simulink model "unitVisualAqSurveillance"  (R2019b)
settings: Solver=VariableStepAuto  StartTime=0.0  StopTime=10.0  RelTol=1e-3
undefined symbols (not defined in the file or in its folder): ac1dyn_alt0_ft, ac1dyn_con, ac1dyn_lat0_rad, ac1dyn_lon0_rad, ac2dyn_alt0_ft, ac2dyn_con, ac2dyn_lat0_rad, ac2dyn_lon0_rad, ddh_ftps2, dh_ftps, dv_ftps2, e_ft, Edot_ftps, h_ft, hdot_ftps, latLonAltState, n_ft, Ndot_ftps, p_radps, phi_rad, phidot_radps, psi_rad, psidot_radps, q_radps, r_radps, theta_rad, thetadot_radps, v_ftps, vdot_fpss
libraries: simulink x14, VisualAqSurveillanceBlock_devAlt x1
(part 1 of 2)
settings Model: Creator=PE29732  LastModifiedBy=ng21251
settings DataIOCC: ReturnWorkspaceOutputs=off
settings DebuggingCC: ArithmeticOperatorsInVariantConditions=warning
settings SFSimCC: CustomCodeUndefinedFunction=UseInterfaceOnly

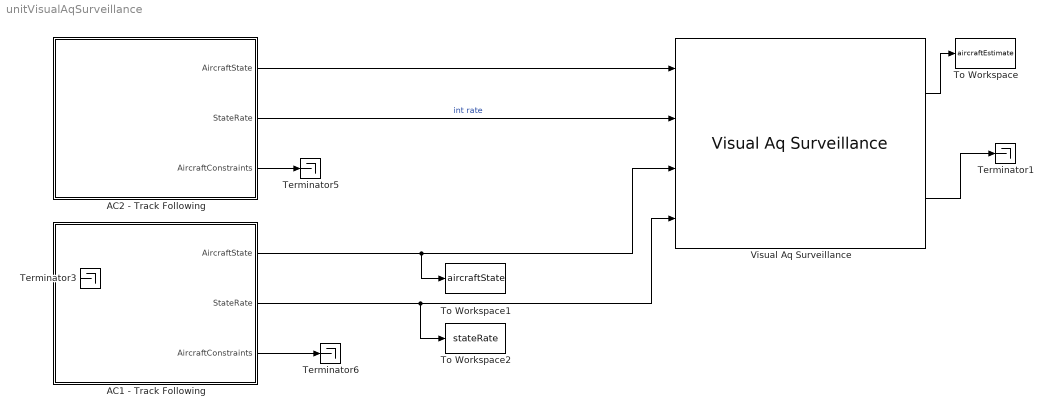
== system unitVisualAqSurveillance ==
  AC1 - Track Following : Subsystem  mask(Basic Aircraft Dynamic Model){ts_dynamics=0.1, lat0_rad=ac1dyn_lat0_rad, lon0_rad=ac1dyn_lon0_rad, alt_ft=ac1dyn_alt0_ft, v_ftps_max=ac1dyn_con.maxAirspeed_ftps, v_ftps_min=ac1dyn_con.minAirspeed_ftps, dv_ftpss_max=ac1dyn_con.maxAcceleration_ftpss, dv_ftpss_min=ac1dyn_con.minAcceleration_ftpss, dh_ftps_max=ac1dyn_con.maxVerticalRate_ftps, dh_ftps_min=ac1dyn_con.minVerticalRate_ftps, q_radps_max=ac1dyn_con.maxPitchRate_radps, phi_rad_max=ac1dyn_con.maxBankAngle_rad, dphi_radps_max=ac1dyn_con.maxRollRate_radps, r_radps_max=ac1dyn_con.maxYawRate_radps, pNUM=ac1dyn_con.dynamicsNumeratorRollRate, pDEN=ac1dyn_con.dynamicsDenominatorRollRate, hNUM=ac1dyn_con.dynamicsNumeratorVerticalRate, hDEN=ac1dyn_con.dynamicsDenominatorVerticalRate, rNUM=ac1dyn_con.dynamicsNumeratorYawRate, rDEN=ac1dyn_con.dynamicsDenominatorYawRate}
      mask prompts: ts_dynamics "Dynamics update parameter"; lat0_rad "Latitude of ENU origin (rad)"; lon0_rad "Longitude of ENU origin (rad)"; alt_ft "Height of ENU origin (ft)"; v_ftps_max "Maximum airspeed (ft/s)"; v_ftps_min "Minimum airspeed (ft/s)"; dv_ftpss_max "Maximum acceleration (ft/s/s)"; dv_ftpss_min "Miniimum acceleration (ft/s/s)"; dh_ftps_max "Maximum vertical rate (ft/s)"; dh_ftps_min "Minimum vertical rate (ft/s)"; q_radps_max "Maximum pitch rate (rad/s)"; phi_rad_max "Maximum bank angle (rad)"; dphi_radps_max "Maximum roll rate (rad/s)"; r_radps_max "Maximum yaw rate (rad/s)"; pNUM "Roll rate discrete dynamics numerator (2x1)"; pDEN "Roll rate discrete dynamics denominator (1x1)"; hNUM "Vertical rate discrete dynamics numerator (2x1)"; hDEN "Vertical rate discrete dynamics denominator (1x1)"; rNUM "Yaw rate discrete dynamics numerator (2x1)"; rDEN "Yaw rate discrete dynamics denominator (1x1)"
      mask help:
      | Propagates the aircraft dynamics using 6DOF equations of motion.
      |
      | The class Simple6DOF can be used to programmatically set the parameters of Basic Aircraft Dynamcis blocks.
      mask Help:
      | Propagates the aircraft dynamics using 6DOF equations of motion.
      | 
      | The class Simple6DOF can be used to programmatically set the parameters of Basic Aircraft Dynamcis blocks.
      mask DialogControl ParameterTabVar0 Prompt: Main
      mask DialogControl ParameterTabVar01 Prompt: Constraints
  AC2 - Track Following : Subsystem  mask(Basic Aircraft Dynamic Model){ts_dynamics=0.1, lat0_rad=ac2dyn_lat0_rad, lon0_rad=ac2dyn_lon0_rad, alt_ft=ac2dyn_alt0_ft, v_ftps_max=ac2dyn_con.maxAirspeed_ftps, v_ftps_min=ac2dyn_con.minAirspeed_ftps, dv_ftpss_max=ac2dyn_con.maxAcceleration_ftpss, dv_ftpss_min=ac2dyn_con.minAcceleration_ftpss, dh_ftps_max=ac2dyn_con.maxVerticalRate_ftps, dh_ftps_min=ac2dyn_con.minVerticalRate_ftps, q_radps_max=ac2dyn_con.maxPitchRate_radps, phi_rad_max=ac2dyn_con.maxBankAngle_rad, dphi_radps_max=ac2dyn_con.maxRollRate_radps, r_radps_max=ac2dyn_con.maxYawRate_radps, pNUM=ac2dyn_con.dynamicsNumeratorRollRate, pDEN=ac2dyn_con.dynamicsDenominatorRollRate, hNUM=ac2dyn_con.dynamicsNumeratorVerticalRate, hDEN=ac2dyn_con.dynamicsDenominatorVerticalRate, rNUM=ac2dyn_con.dynamicsNumeratorYawRate, rDEN=ac2dyn_con.dynamicsDenominatorYawRate}
      mask prompts: ts_dynamics "Dynamics update parameter"; lat0_rad "Latitude of ENU origin (rad)"; lon0_rad "Longitude of ENU origin (rad)"; alt_ft "Height of ENU origin (ft)"; v_ftps_max "Maximum airspeed (ft/s)"; v_ftps_min "Minimum airspeed (ft/s)"; dv_ftpss_max "Maximum acceleration (ft/s/s)"; dv_ftpss_min "Miniimum acceleration (ft/s/s)"; dh_ftps_max "Maximum vertical rate (ft/s)"; dh_ftps_min "Minimum vertical rate (ft/s)"; q_radps_max "Maximum pitch rate (rad/s)"; phi_rad_max "Maximum bank angle (rad)"; dphi_radps_max "Maximum roll rate (rad/s)"; r_radps_max "Maximum yaw rate (rad/s)"; pNUM "Roll rate discrete dynamics numerator (2x1)"; pDEN "Roll rate discrete dynamics denominator (1x1)"; hNUM "Vertical rate discrete dynamics numerator (2x1)"; hDEN "Vertical rate discrete dynamics denominator (1x1)"; rNUM "Yaw rate discrete dynamics numerator (2x1)"; rDEN "Yaw rate discrete dynamics denominator (1x1)"
      mask help:
      | Propagates the aircraft dynamics using 6DOF equations of motion.
      |
      | The class Simple6DOF can be used to programmatically set the parameters of Basic Aircraft Dynamcis blocks.
      mask Help:
      | Propagates the aircraft dynamics using 6DOF equations of motion.
      | 
      | The class Simple6DOF can be used to programmatically set the parameters of Basic Aircraft Dynamcis blocks.
      mask DialogControl ParameterTabVar0 Prompt: Main
      mask DialogControl ParameterTabVar01 Prompt: Constraints
  Terminator{1,3,5..6} (4 alike) : Terminator
  To Workspace : ToWorkspace  VariableName=aircraftEstimate  SaveFormat=Timeseries  SampleTime=-1
  To Workspace1 : ToWorkspace  VariableName=aircraftState  SaveFormat=Timeseries  SampleTime=-1
  To Workspace2 : ToWorkspace  VariableName=stateRate  SaveFormat=Timeseries  SampleTime=-1
  Visual Aq Surveillance : VisualAqSurveillanceBlock_devAlt/Visual Aq Surveillance  Description=|  dt=0.1
      | Documentation for Perfect Observation Block                                                                                                                                                                                                                                                                                                                                                                                                          
      |                                                                                                                                                                                                                                                                                                                                                                                                                                                      
      | Description:  The perfect observation block, also known as a perfect                                                                                                                                                                                                                                                                                                                                                                                 
      | surveillance block, receives an Aircraft State, nominally from a Basic                                                                                                                                                                                                                                                                                                                                                                               
      | Aircraft Dynamics block, and outputs an Aircraft Estimate.  The Aircraft                                                                                                                                                                                                                                                                                                                                                                             
      | State that is received as input consists of Latitude, Longitude, and                                                                                                                                                                                                                                                                                                                                                                                 
      | Altitude state information as well as the aircraft position in local                                                                                                                                                                                                                                                                                                                                                                                 
      | coordinates in units of feet for north, east, and height.  The Aircraft                                                                                                                                                                                                                                                                                                                                                                              
      | Estimate outputs consist of estimates for the aircraft Latitude, Longitude, and Altitude, the east, north up position, and sensor covariance.  For perfect surveillance, the covariance estimates are all set to zero as default.  In addition, "time of validity" and a Boolean flag for the sensor report, "is Valid", are outputted as part of the Aircraft Estimate.                                                                             
      |                                                                                                                                                                                                                                                                                                                                                                                                                                                      
      | The initial perfect surveillance block developed receives the aircraft state information from the "AC2 - Basic Aircraft Dynamics" block within the "nominalEncounter" study.  Since the expected output from the AC1 and AC2 aircraft states have slightly different output parameters than what is provided from the perfect surveillance block (i.e., covariance estimates, isValid, and time of validity), the perfect surveillance block         
      | AircraftEstimate output has been left disconnected.                                                                                                                                                                                                                                                                                                                                                                                                  
      |                                                                                                                                                                                                                                                                                                                                                                                                                                                      
      | The initial unit test performed for this perfect observation block was to                                                                                                                                                                                                                                                                                                                                                                            
      | run the nominalEncounter study and to ensure that the simulation completes and no exceptions are encountered.  This unit test was successful (other than receiving a warning that the output of the perfect surveillance block is not connected, which was expected).  A more comprehensive future unit test would be to evaluate the position inputs and compare them with the position outputs to ensure that they are consistent with one another.
  wires:
  AC1 - Track Following/1(AircraftState) -> Visual Aq Surveillance/3, To Workspace1/1
  Visual Aq Surveillance/1 -> To Workspace/1
  Visual Aq Surveillance/2 -> Terminator1/1
  AC1 - Track Following/2(StateRate) -> Visual Aq Surveillance/4, To Workspace2/1
  AC2 - Track Following/1(AircraftState) -> Visual Aq Surveillance/1
  AC2 - Track Following/3(AircraftConstraints) -> Terminator5/1
  AC1 - Track Following/3(AircraftConstraints) -> Terminator6/1
  AC2 - Track Following/2(StateRate) -> Visual Aq Surveillance/2  "int rate"

== system unitVisualAqSurveillance/AC1 - Track Following ==
  Follow Trajectory : Subsystem  mask(Follow Trajectory){trajfile=traj1.mat}
      mask prompts: trajfile "Trajectory File Name:"
      mask help: Reads trajectory data (North-East-Altitude position and velocity) from specified file. Computes other state variables to follow that trajectory. Ouptuts AircraftState and AircraftStateRate buses.
      mask init:
      | set_param( [ gcb '/Get Trajectory Data/From File' ], 'Filename', trajfile )
  Performance_constraints : Subsystem
  Rate Transition : RateTransition  OutPortSampleTime=0.1
  AircraftState : Outport  OutDataTypeStr=Bus: AircraftState  VectorParamsAs1DForOutWhenUnconnected=off
  StateRate : Outport  Port=2  OutDataTypeStr=Bus: AircraftStateRate  VectorParamsAs1DForOutWhenUnconnected=off
  AircraftConstraints : Outport  Port=3  OutDataTypeStr=Bus: AircraftConstraints  VectorParamsAs1DForOutWhenUnconnected=off
  wires:
  Follow Trajectory/2(State Rate) -> Rate Transition/1
  Follow Trajectory/1(State) -> AircraftState/1
  Performance_constraints/1(AircraftConstraints) -> Follow Trajectory/1(Constraints), AircraftConstraints/1
  Rate Transition/1 -> StateRate/1

== system unitVisualAqSurveillance/AC2 - Track Following ==
  Follow Trajectory : Subsystem  mask(Follow Trajectory){trajfile=traj2.mat}
      mask prompts: trajfile "Trajectory File Name:"
      mask help: Reads trajectory data (North-East-Altitude position and velocity) from specified file. Computes other state variables to follow that trajectory. Ouptuts AircraftState and AircraftStateRate buses.
      mask init:
      | set_param( [ gcb '/Get Trajectory Data/From File' ], 'Filename', trajfile )
  Performance_constraints : Subsystem
  Rate Transition : RateTransition  OutPortSampleTime=0.1
  AircraftState : Outport  OutDataTypeStr=Bus: AircraftState  VectorParamsAs1DForOutWhenUnconnected=off
  StateRate : Outport  Port=2  OutDataTypeStr=Bus: AircraftStateRate  VectorParamsAs1DForOutWhenUnconnected=off
  AircraftConstraints : Outport  Port=3  OutDataTypeStr=Bus: AircraftConstraints  VectorParamsAs1DForOutWhenUnconnected=off
  wires:
  Follow Trajectory/2(State Rate) -> Rate Transition/1
  Follow Trajectory/1(State) -> AircraftState/1
  Performance_constraints/1(AircraftConstraints) -> Follow Trajectory/1(Constraints), AircraftConstraints/1
  Rate Transition/1 -> StateRate/1

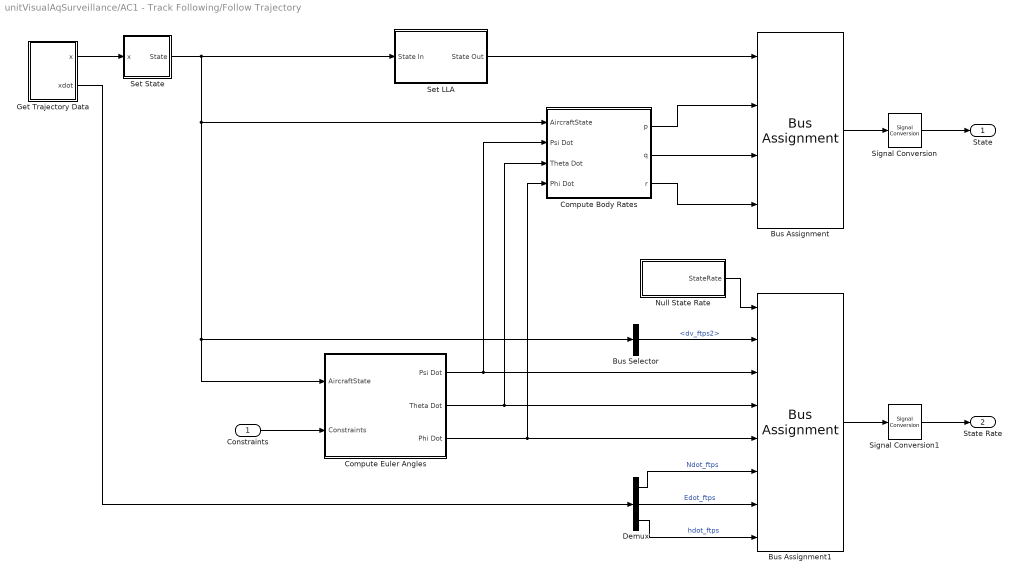
== system unitVisualAqSurveillance/AC1 - Track Following/Follow Trajectory ==
  Constraints : Inport
  Bus Assignment : BusAssignment  AssignedSignals=p_radps,q_radps,r_radps
  Bus Assignment1 : BusAssignment  AssignedSignals=vdot_fpss,psidot_radps,thetadot_radps,phidot_radps,Ndot_ftps,Edot_ftps,hdot_ftps
  Bus Selector : BusSelector  OutputSignals=dv_ftps2
  Compute Body Rates : Subsystem
  Compute Euler Angles : Subsystem
  Demux : Demux  Outputs=3
  Get Trajectory Data : Subsystem
  Null State Rate : Subsystem
  "Set LLA " : Subsystem  mask{lat0=lat0_rad, lon0=lon0_rad, h0=alt_ft}
      mask prompts: lat0 "ENU latitude origin (rad)"; lon0 "ENU longitude origin (rad)"; h0 "ENU altitude origin (ft)"
  Set State : Subsystem
  Signal Conversion : SignalConversion  OverrideOpt=off
  Signal Conversion1 : SignalConversion  OverrideOpt=off
  State : Outport  VectorParamsAs1DForOutWhenUnconnected=off
  State Rate : Outport  Port=2  VectorParamsAs1DForOutWhenUnconnected=off
  wires:
  Signal Conversion1/1 -> State Rate/1
  Bus Selector/1 -> Bus Assignment1/2  "<dv_ftps2>"
  Compute Euler Angles/3("Phi Dot ") -> Bus Assignment1/5, Compute Body Rates/4(Phi Dot)
  Compute Euler Angles/1(Psi Dot) -> Bus Assignment1/3, Compute Body Rates/2(Psi Dot)
  Demux/3 -> Bus Assignment1/8  "hdot_ftps"
  Null State Rate/1(StateRate) -> Bus Assignment1/1
  Get Trajectory Data/2(xdot) -> Demux/1
  Compute Body Rates/3(r) -> Bus Assignment/4
  Compute Body Rates/2(q) -> Bus Assignment/3
  Compute Body Rates/1(p) -> Bus Assignment/2
  Demux/1 -> Bus Assignment1/6  "Ndot_ftps"
  Demux/2 -> Bus Assignment1/7  "Edot_ftps"
  Compute Euler Angles/2(Theta Dot) -> Bus Assignment1/4, Compute Body Rates/3(Theta Dot)
  Signal Conversion/1 -> State/1
  "Set LLA "/1(State Out) -> Bus Assignment/1
  Bus Assignment/1 -> Signal Conversion/1
  Bus Assignment1/1 -> Signal Conversion1/1
  Set State/1(State) -> Compute Body Rates/1(AircraftState), Compute Euler Angles/1(AircraftState), Bus Selector/1, "Set LLA "/1(State In)
  Constraints/1 -> Compute Euler Angles/2(Constraints)
  Get Trajectory Data/1(x) -> Set State/1(x)

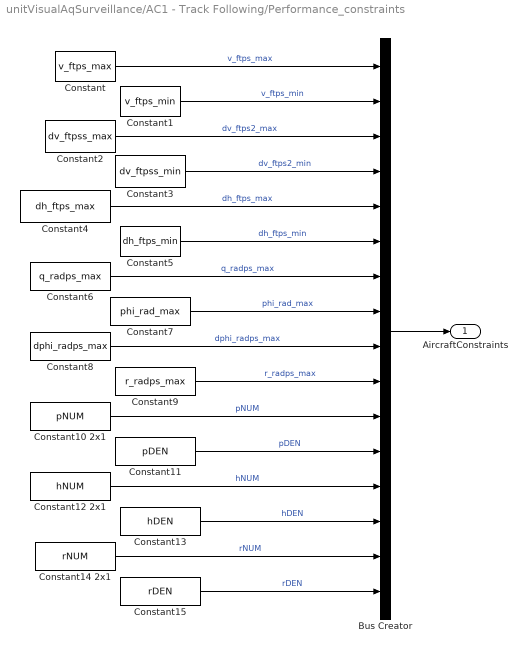
== system unitVisualAqSurveillance/AC1 - Track Following/Performance_constraints ==
  Bus Creator : BusCreator  Inputs=16
  Constant : Constant  Value=v_ftps_max
  Constant1 : Constant  Value=v_ftps_min
  Constant10 2x1 : Constant  Value=pNUM
  Constant11 : Constant  Value=pDEN
  Constant12 2x1 : Constant  Value=hNUM
  Constant13 : Constant  Value=hDEN
  Constant14 2x1 : Constant  Value=rNUM
  Constant15 : Constant  Value=rDEN
  Constant2 : Constant  Value=dv_ftpss_max
  Constant3 : Constant  Value=dv_ftpss_min
  Constant4 : Constant  Value=dh_ftps_max
  Constant5 : Constant  Value=dh_ftps_min
  Constant6 : Constant  Value=q_radps_max
  Constant7 : Constant  Value=phi_rad_max
  Constant8 : Constant  Value=dphi_radps_max
  Constant9 : Constant  Value=r_radps_max
  AircraftConstraints : Outport  OutDataTypeStr=Bus: AircraftConstraints  VectorParamsAs1DForOutWhenUnconnected=off
  wires:
  Constant10 2x1/1 -> Bus Creator/11  "pNUM"
  Constant12 2x1/1 -> Bus Creator/13  "hNUM"
  Constant14 2x1/1 -> Bus Creator/15  "rNUM"
  Constant8/1 -> Bus Creator/9  "dphi_radps_max"
  Constant7/1 -> Bus Creator/8  "phi_rad_max"
  Constant6/1 -> Bus Creator/7  "q_radps_max"
  Constant5/1 -> Bus Creator/6  "dh_ftps_min"
  Constant4/1 -> Bus Creator/5  "dh_ftps_max"
  Constant3/1 -> Bus Creator/4  "dv_ftps2_min"
  Constant2/1 -> Bus Creator/3  "dv_ftps2_max"
  Constant1/1 -> Bus Creator/2  "v_ftps_min"
  Constant/1 -> Bus Creator/1  "v_ftps_max"
  Bus Creator/1 -> AircraftConstraints/1
  Constant15/1 -> Bus Creator/16  "rDEN"
  Constant13/1 -> Bus Creator/14  "hDEN"
  Constant11/1 -> Bus Creator/12  "pDEN"
  Constant9/1 -> Bus Creator/10  "r_radps_max"

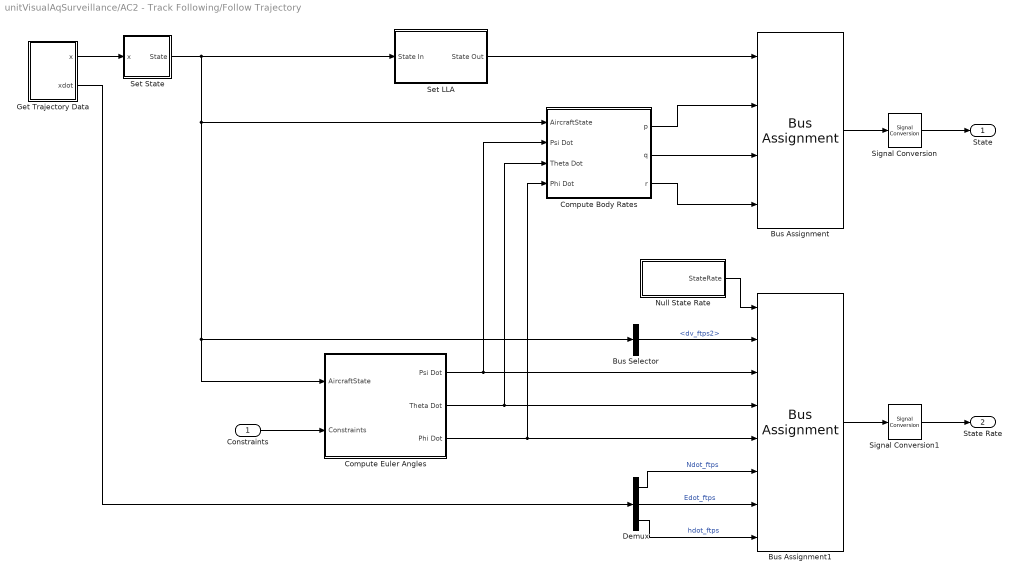
== system unitVisualAqSurveillance/AC2 - Track Following/Follow Trajectory ==
  Constraints : Inport
  Bus Assignment : BusAssignment  AssignedSignals=p_radps,q_radps,r_radps
  Bus Assignment1 : BusAssignment  AssignedSignals=vdot_fpss,psidot_radps,thetadot_radps,phidot_radps,Ndot_ftps,Edot_ftps,hdot_ftps
  Bus Selector : BusSelector  OutputSignals=dv_ftps2
  Compute Body Rates : Subsystem
  Compute Euler Angles : Subsystem
  Demux : Demux  Outputs=3
  Get Trajectory Data : Subsystem
  Null State Rate : Subsystem
  "Set LLA " : Subsystem  mask{lat0=lat0_rad, lon0=lon0_rad, h0=alt_ft}
      mask prompts: lat0 "ENU latitude origin (rad)"; lon0 "ENU longitude origin (rad)"; h0 "ENU altitude origin (ft)"
  Set State : Subsystem
  Signal Conversion : SignalConversion  OverrideOpt=off
  Signal Conversion1 : SignalConversion  OverrideOpt=off
  State : Outport  VectorParamsAs1DForOutWhenUnconnected=off
  State Rate : Outport  Port=2  VectorParamsAs1DForOutWhenUnconnected=off
  wires:
  Signal Conversion1/1 -> State Rate/1
  Bus Selector/1 -> Bus Assignment1/2  "<dv_ftps2>"
  Compute Euler Angles/3("Phi Dot ") -> Bus Assignment1/5, Compute Body Rates/4(Phi Dot)
  Compute Euler Angles/1(Psi Dot) -> Bus Assignment1/3, Compute Body Rates/2(Psi Dot)
  Demux/3 -> Bus Assignment1/8  "hdot_ftps"
  Null State Rate/1(StateRate) -> Bus Assignment1/1
  Get Trajectory Data/2(xdot) -> Demux/1
  Compute Body Rates/3(r) -> Bus Assignment/4
  Compute Body Rates/2(q) -> Bus Assignment/3
  Compute Body Rates/1(p) -> Bus Assignment/2
  Demux/1 -> Bus Assignment1/6  "Ndot_ftps"
  Demux/2 -> Bus Assignment1/7  "Edot_ftps"
  Compute Euler Angles/2(Theta Dot) -> Bus Assignment1/4, Compute Body Rates/3(Theta Dot)
  Signal Conversion/1 -> State/1
  "Set LLA "/1(State Out) -> Bus Assignment/1
  Bus Assignment/1 -> Signal Conversion/1
  Bus Assignment1/1 -> Signal Conversion1/1
  Set State/1(State) -> Compute Body Rates/1(AircraftState), Compute Euler Angles/1(AircraftState), Bus Selector/1, "Set LLA "/1(State In)
  Constraints/1 -> Compute Euler Angles/2(Constraints)
  Get Trajectory Data/1(x) -> Set State/1(x)

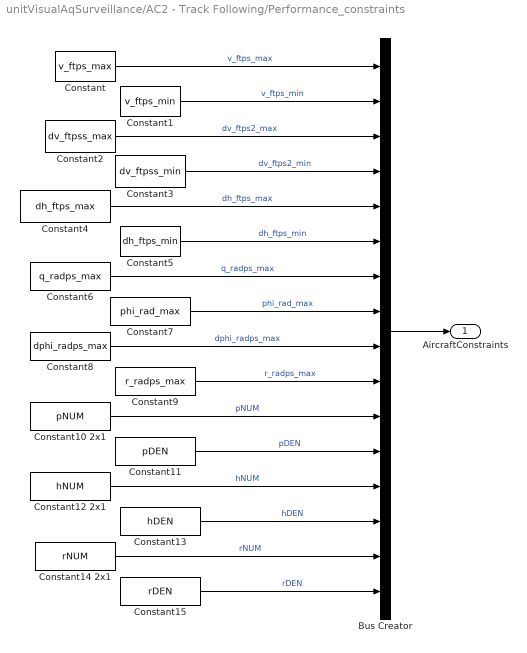
== system unitVisualAqSurveillance/AC2 - Track Following/Performance_constraints ==
  Bus Creator : BusCreator  Inputs=16
  Constant : Constant  Value=v_ftps_max
  Constant1 : Constant  Value=v_ftps_min
  Constant10 2x1 : Constant  Value=pNUM
  Constant11 : Constant  Value=pDEN
  Constant12 2x1 : Constant  Value=hNUM
  Constant13 : Constant  Value=hDEN
  Constant14 2x1 : Constant  Value=rNUM
  Constant15 : Constant  Value=rDEN
  Constant2 : Constant  Value=dv_ftpss_max
  Constant3 : Constant  Value=dv_ftpss_min
  Constant4 : Constant  Value=dh_ftps_max
  Constant5 : Constant  Value=dh_ftps_min
  Constant6 : Constant  Value=q_radps_max
  Constant7 : Constant  Value=phi_rad_max
  Constant8 : Constant  Value=dphi_radps_max
  Constant9 : Constant  Value=r_radps_max
  AircraftConstraints : Outport  OutDataTypeStr=Bus: AircraftConstraints  VectorParamsAs1DForOutWhenUnconnected=off
  wires:
  Constant10 2x1/1 -> Bus Creator/11  "pNUM"
  Constant12 2x1/1 -> Bus Creator/13  "hNUM"
  Constant14 2x1/1 -> Bus Creator/15  "rNUM"
  Constant8/1 -> Bus Creator/9  "dphi_radps_max"
  Constant7/1 -> Bus Creator/8  "phi_rad_max"
  Constant6/1 -> Bus Creator/7  "q_radps_max"
  Constant5/1 -> Bus Creator/6  "dh_ftps_min"
  Constant4/1 -> Bus Creator/5  "dh_ftps_max"
  Constant3/1 -> Bus Creator/4  "dv_ftps2_min"
  Constant2/1 -> Bus Creator/3  "dv_ftps2_max"
  Constant1/1 -> Bus Creator/2  "v_ftps_min"
  Constant/1 -> Bus Creator/1  "v_ftps_max"
  Bus Creator/1 -> AircraftConstraints/1
  Constant15/1 -> Bus Creator/16  "rDEN"
  Constant13/1 -> Bus Creator/14  "hDEN"
  Constant11/1 -> Bus Creator/12  "pDEN"
  Constant9/1 -> Bus Creator/10  "r_radps_max"

== system unitVisualAqSurveillance/AC1 - Track Following/Follow Trajectory/Compute Body Rates ==
  AircraftState : Inport
  Psi Dot : Inport  Port=2
  Theta Dot : Inport  Port=3
  Phi Dot : Inport  Port=4
  Bus Creator : BusCreator  Inputs=3
  Compute p : Subsystem
  Compute q : Subsystem
  Compute r : Subsystem
  p : Outport  VectorParamsAs1DForOutWhenUnconnected=off
  q : Outport  Port=2  VectorParamsAs1DForOutWhenUnconnected=off
  r : Outport  Port=3  VectorParamsAs1DForOutWhenUnconnected=off
  wires:
  Compute r/1(r) -> r/1
  Compute q/1(q) -> q/1
  Compute p/1(p) -> p/1
  Bus Creator/1 -> Compute p/2(Euler Rates), Compute q/2(Euler Rates), Compute r/2(Euler Rates)
  AircraftState/1 -> Compute p/1(State), Compute q/1(State), Compute r/1(State)
  Psi Dot/1 -> Bus Creator/1  "psidot"
  Phi Dot/1 -> Bus Creator/3  "phidot"
  Theta Dot/1 -> Bus Creator/2  "thetadot"

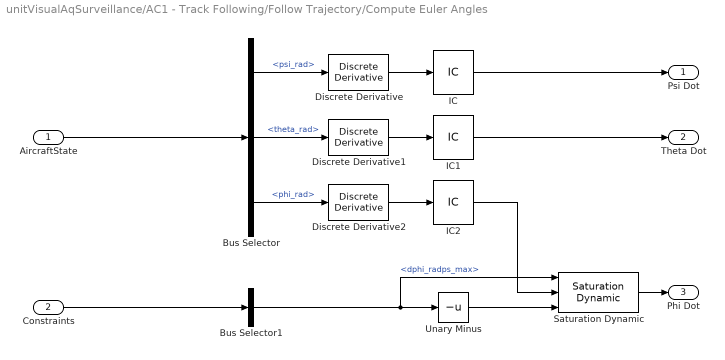
== system unitVisualAqSurveillance/AC1 - Track Following/Follow Trajectory/Compute Euler Angles ==
  AircraftState : Inport
  Constraints : Inport  Port=2
  Bus Selector : BusSelector  OutputSignals=psi_rad,theta_rad,phi_rad
  Bus Selector1 : BusSelector  OutputSignals=dphi_radps_max
  Discrete Derivative : simulink/Discrete/Discrete Derivative  gainval=1.0  ICPrevScaledInput=0.0  OutMin=[]  OutMax=[]  OutDataType=fixdt(1, 16)  OutScaling=2^-10  DoSatur=off
  Discrete Derivative1 : simulink/Discrete/Discrete Derivative  gainval=1.0  ICPrevScaledInput=0.0  OutMin=[]  OutMax=[]  OutDataType=fixdt(1, 16)  OutScaling=2^-10  DoSatur=off
  Discrete Derivative2 : simulink/Discrete/Discrete Derivative  gainval=1.0  ICPrevScaledInput=0.0  OutMin=[]  OutMax=[]  OutDataType=fixdt(1, 16)  OutScaling=2^-10  DoSatur=off
  IC : InitialCondition  Value=0
  IC1 : InitialCondition  Value=0
  IC2 : InitialCondition  Value=0
  Saturation Dynamic : simulink/Discontinuities/Saturation Dynamic  OutMin=[]  OutMax=[]  OutDataTypeStr=Inherit: Same as second input  OutDataType=fixdt(1, 16)  OutScaling=2^-10  DoSatur=off
  Unary Minus : UnaryMinus
  Psi Dot : Outport  VectorParamsAs1DForOutWhenUnconnected=off
  Theta Dot : Outport  Port=2  VectorParamsAs1DForOutWhenUnconnected=off
  "Phi Dot " : Outport  Port=3  VectorParamsAs1DForOutWhenUnconnected=off
  wires:
  Constraints/1 -> Bus Selector1/1
  IC2/1 -> Saturation Dynamic/2
  IC1/1 -> Theta Dot/1
  IC/1 -> Psi Dot/1
  Discrete Derivative2/1 -> IC2/1
  Discrete Derivative1/1 -> IC1/1
  Discrete Derivative/1 -> IC/1
  Bus Selector/3 -> Discrete Derivative2/1  "<phi_rad>"
  Bus Selector/2 -> Discrete Derivative1/1  "<theta_rad>"
  Bus Selector/1 -> Discrete Derivative/1  "<psi_rad>"
  AircraftState/1 -> Bus Selector/1
  Saturation Dynamic/1 -> "Phi Dot "/1
  Bus Selector1/1 -> Unary Minus/1, Saturation Dynamic/1  "<dphi_radps_max>"
  Unary Minus/1 -> Saturation Dynamic/3

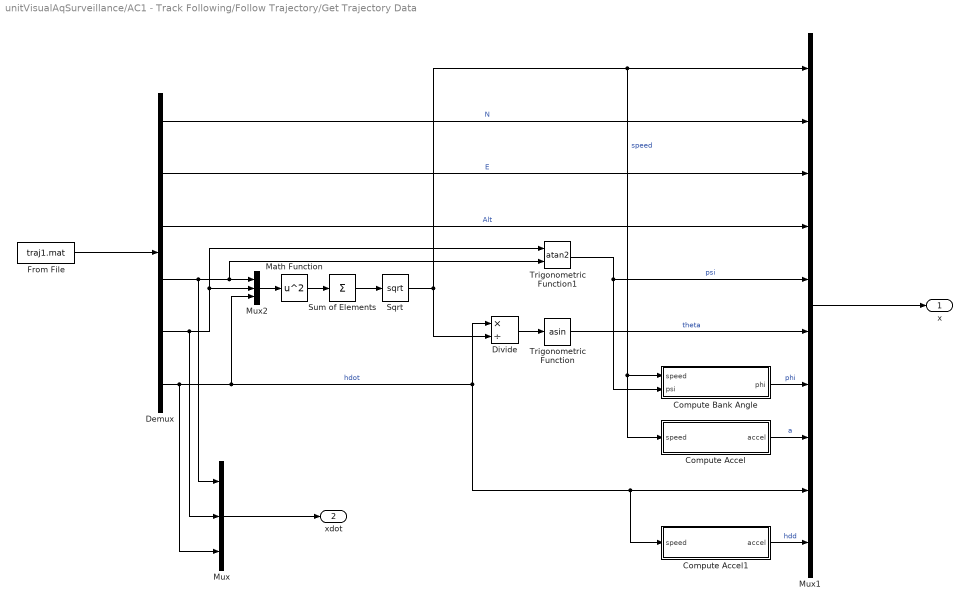
== system unitVisualAqSurveillance/AC1 - Track Following/Follow Trajectory/Get Trajectory Data ==
  Compute Accel : Subsystem
  Compute Accel1 : Subsystem
  Compute Bank Angle : Subsystem
  Demux : Demux  Outputs=6
  Divide : Product  Inputs=*/
  From File : FromFile  FileName=traj1.mat  SampleTime=0.1
  Math Function : Math  Operator=square  SaturateOnIntegerOverflow=on
  Mux : Mux  Inputs=3
  Mux1 : Mux  Inputs=10
  Mux2 : Mux  Inputs=3
  Sqrt : Sqrt  SaturateOnIntegerOverflow=on
  Sum of Elements : Sum  Inputs=+
  Trigonometric Function : Trigonometry  Operator=asin
  Trigonometric Function1 : Trigonometry  Operator=atan2
  x : Outport  VectorParamsAs1DForOutWhenUnconnected=off
  xdot : Outport  Port=2  VectorParamsAs1DForOutWhenUnconnected=off
  wires:
  Mux/1 -> xdot/1
  Compute Accel1/1(accel) -> Mux1/10  "hdd"
  Demux/5 -> Mux2/2, Trigonometric Function1/1, Mux/2
  Divide/1 -> Trigonometric Function/1
  Trigonometric Function1/1 -> Mux1/5, Compute Bank Angle/2(psi)  "psi"
  Trigonometric Function/1 -> Mux1/6  "theta"
  Compute Bank Angle/1(phi) -> Mux1/7  "phi"
  Compute Accel/1(accel) -> Mux1/8  "a"
  Mux1/1 -> x/1
  Sqrt/1 -> Divide/2, Mux1/1, Compute Bank Angle/1(speed), Compute Accel/1(speed)  "speed"
  Sum of Elements/1 -> Sqrt/1
  Math Function/1 -> Sum of Elements/1
  Mux2/1 -> Math Function/1
  Demux/6 -> Mux1/9, Compute Accel1/1(speed), Divide/1, Mux2/3, Mux/3  "hdot"
  Demux/4 -> Mux2/1, Trigonometric Function1/2, Mux/1
  Demux/3 -> Mux1/4  "Alt"
  Demux/2 -> Mux1/3  "E"
  Demux/1 -> Mux1/2  "N"
  From File/1 -> Demux/1

== system unitVisualAqSurveillance/AC1 - Track Following/Follow Trajectory/Null State Rate ==
  Bus Creator : BusCreator  Inputs='vdot_fpss','Ndot_ftps','Edot_ftps','hdot_ftps','psidot_radps','thetadot_radps','phidot_radps'  OutDataTypeStr=Bus: AircraftStateRate
  Constant{,1..6} (7 alike) : Constant  Value=0
  StateRate : Outport  OutDataTypeStr=Bus: AircraftStateRate  VectorParamsAs1DForOutWhenUnconnected=off
  wires:
  Constant6/1 -> Bus Creator/7  "phidot_radps"
  Constant5/1 -> Bus Creator/6  "thetadot_radps"
  Constant4/1 -> Bus Creator/5  "psidot_radps"
  Constant3/1 -> Bus Creator/4  "hdot_ftps"
  Constant2/1 -> Bus Creator/3  "Edot_ftps"
  Constant1/1 -> Bus Creator/2  "Ndot_ftps"
  Constant/1 -> Bus Creator/1  "vdot_fpss"
  Bus Creator/1 -> StateRate/1

== system unitVisualAqSurveillance/AC1 - Track Following/Follow Trajectory/Set LLA  ==
  State In : Inport
  Bus Assignment : BusAssignment  AssignedSignals=latLonAltState.lat_rad,latLonAltState.lon_rad,latLonAltState.dlat_radps,latLonAltState.dlon_radps,latLonAltState.alt_ft,latLonAltState.dalt_ftps
  Bus Selector : BusSelector  OutputSignals=e_ft,n_ft,h_ft,v_ftps,psi_rad,theta_rad
  Constant : Constant  Value=lat0
  Constant7 : Constant  Value=lon0
  Constant8 : Constant  Value=h0
  MATLAB Function : MATLAB Function  TreatAsAtomicUnit=on
  State Out : Outport  VectorParamsAs1DForOutWhenUnconnected=off
  wires:
  Bus Selector/6 -> MATLAB Function/6(theta_rad)  "<theta_rad>"
  Bus Selector/5 -> MATLAB Function/5(psi_rad)  "<psi_rad>"
  Bus Selector/4 -> MATLAB Function/4(v_ftps)  "<v_ftps>"
  Bus Selector/3 -> MATLAB Function/3(u_ft)  "<h_ft>"
  Bus Selector/2 -> MATLAB Function/2(n_ft)  "<n_ft>"
  Bus Selector/1 -> MATLAB Function/1(e_ft)  "<e_ft>"
  Constant8/1 -> MATLAB Function/9(h0)
  Constant7/1 -> MATLAB Function/8(lon0)
  Constant/1 -> MATLAB Function/7(lat0)
  State In/1 -> Bus Selector/1, Bus Assignment/1
  Bus Assignment/1 -> State Out/1
  MATLAB Function/6(dalt_ftps) -> Bus Assignment/7  "dalt_ftps"
  MATLAB Function/5(alt_ft) -> Bus Assignment/6  "alt_ft"
  MATLAB Function/4(dlon_radps) -> Bus Assignment/5  "dlon_radps"
  MATLAB Function/3(dlat_radps) -> Bus Assignment/4  "dlat_radps"
  MATLAB Function/2(lon_rad) -> Bus Assignment/3  "lon_rad"
  MATLAB Function/1(lat_rad) -> Bus Assignment/2  "lat_rad"

== system unitVisualAqSurveillance/AC1 - Track Following/Follow Trajectory/Set State ==
  x : Inport
  Bus Assignment : BusAssignment  AssignedSignals=v_ftps,n_ft,e_ft,h_ft,psi_rad,theta_rad,phi_rad,dv_ftps2,dh_ftps,ddh_ftps2
  Demux : Demux  Outputs=10
  Null AircraftState : Subsystem
  State : Outport  VectorParamsAs1DForOutWhenUnconnected=off
  wires:
  Demux/10 -> Bus Assignment/11
  Demux/9 -> Bus Assignment/10
  Bus Assignment/1 -> State/1
  Null AircraftState/1(State) -> Bus Assignment/1
  Demux/7 -> Bus Assignment/8  "phi"
  x/1 -> Demux/1
  Demux/6 -> Bus Assignment/7  "theta"
  Demux/5 -> Bus Assignment/6  "psi"
  Demux/4 -> Bus Assignment/5  "h"
  Demux/3 -> Bus Assignment/4  "E"
  Demux/2 -> Bus Assignment/3  "N"
  Demux/1 -> Bus Assignment/2  "v"
  Demux/8 -> Bus Assignment/9  "a"

== system unitVisualAqSurveillance/AC2 - Track Following/Follow Trajectory/Compute Body Rates ==
  AircraftState : Inport
  Psi Dot : Inport  Port=2
  Theta Dot : Inport  Port=3
  Phi Dot : Inport  Port=4
  Bus Creator : BusCreator  Inputs=3
  Compute p : Subsystem
  Compute q : Subsystem
  Compute r : Subsystem
  p : Outport  VectorParamsAs1DForOutWhenUnconnected=off
  q : Outport  Port=2  VectorParamsAs1DForOutWhenUnconnected=off
  r : Outport  Port=3  VectorParamsAs1DForOutWhenUnconnected=off
  wires:
  Compute r/1(r) -> r/1
  Compute q/1(q) -> q/1
  Compute p/1(p) -> p/1
  Bus Creator/1 -> Compute p/2(Euler Rates), Compute q/2(Euler Rates), Compute r/2(Euler Rates)
  AircraftState/1 -> Compute p/1(State), Compute q/1(State), Compute r/1(State)
  Psi Dot/1 -> Bus Creator/1  "psidot"
  Phi Dot/1 -> Bus Creator/3  "phidot"
  Theta Dot/1 -> Bus Creator/2  "thetadot"

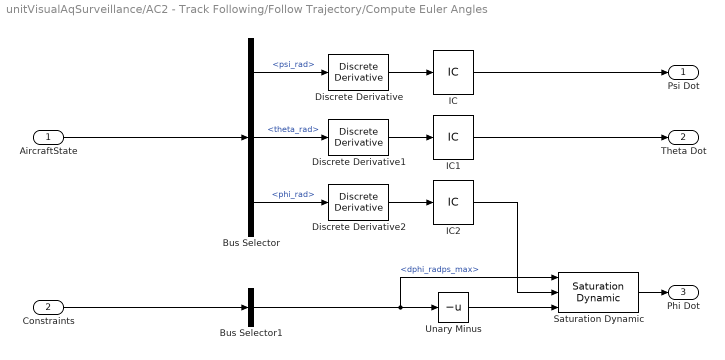
== system unitVisualAqSurveillance/AC2 - Track Following/Follow Trajectory/Compute Euler Angles ==
  AircraftState : Inport
  Constraints : Inport  Port=2
  Bus Selector : BusSelector  OutputSignals=psi_rad,theta_rad,phi_rad
  Bus Selector1 : BusSelector  OutputSignals=dphi_radps_max
  Discrete Derivative : simulink/Discrete/Discrete Derivative  gainval=1.0  ICPrevScaledInput=0.0  OutMin=[]  OutMax=[]  OutDataType=fixdt(1, 16)  OutScaling=2^-10  DoSatur=off
  Discrete Derivative1 : simulink/Discrete/Discrete Derivative  gainval=1.0  ICPrevScaledInput=0.0  OutMin=[]  OutMax=[]  OutDataType=fixdt(1, 16)  OutScaling=2^-10  DoSatur=off
  Discrete Derivative2 : simulink/Discrete/Discrete Derivative  gainval=1.0  ICPrevScaledInput=0.0  OutMin=[]  OutMax=[]  OutDataType=fixdt(1, 16)  OutScaling=2^-10  DoSatur=off
  IC : InitialCondition  Value=0
  IC1 : InitialCondition  Value=0
  IC2 : InitialCondition  Value=0
  Saturation Dynamic : simulink/Discontinuities/Saturation Dynamic  OutMin=[]  OutMax=[]  OutDataTypeStr=Inherit: Same as second input  OutDataType=fixdt(1, 16)  OutScaling=2^-10  DoSatur=off
  Unary Minus : UnaryMinus
  Psi Dot : Outport  VectorParamsAs1DForOutWhenUnconnected=off
  Theta Dot : Outport  Port=2  VectorParamsAs1DForOutWhenUnconnected=off
  "Phi Dot " : Outport  Port=3  VectorParamsAs1DForOutWhenUnconnected=off
  wires:
  Constraints/1 -> Bus Selector1/1
  IC2/1 -> Saturation Dynamic/2
  IC1/1 -> Theta Dot/1
  IC/1 -> Psi Dot/1
  Discrete Derivative2/1 -> IC2/1
  Discrete Derivative1/1 -> IC1/1
  Discrete Derivative/1 -> IC/1
  Bus Selector/3 -> Discrete Derivative2/1  "<phi_rad>"
  Bus Selector/2 -> Discrete Derivative1/1  "<theta_rad>"
  Bus Selector/1 -> Discrete Derivative/1  "<psi_rad>"
  AircraftState/1 -> Bus Selector/1
  Saturation Dynamic/1 -> "Phi Dot "/1
  Bus Selector1/1 -> Unary Minus/1, Saturation Dynamic/1  "<dphi_radps_max>"
  Unary Minus/1 -> Saturation Dynamic/3

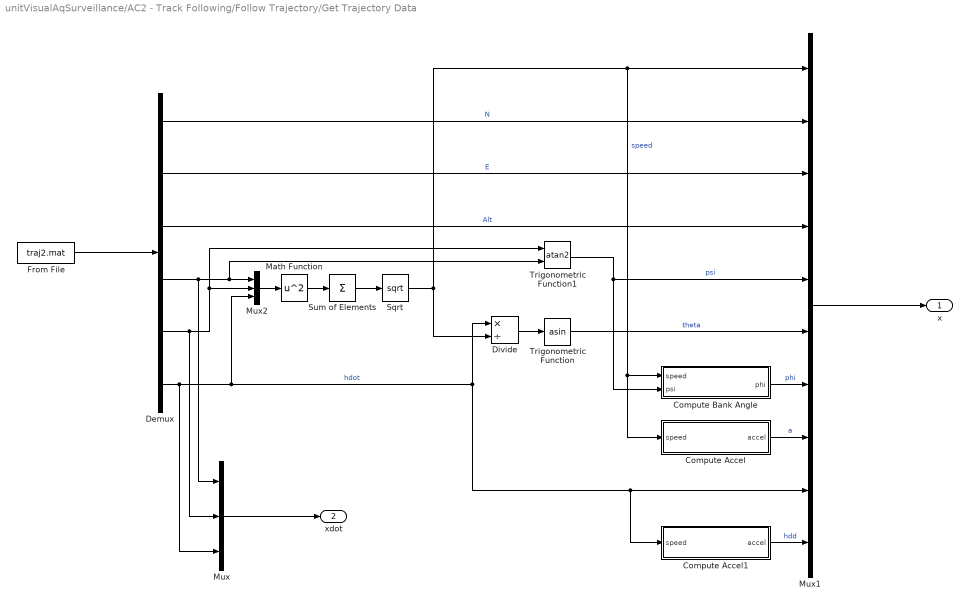
== system unitVisualAqSurveillance/AC2 - Track Following/Follow Trajectory/Get Trajectory Data ==
  Compute Accel : Subsystem
  Compute Accel1 : Subsystem
  Compute Bank Angle : Subsystem
  Demux : Demux  Outputs=6
  Divide : Product  Inputs=*/
  From File : FromFile  FileName=traj2.mat  SampleTime=0.1
  Math Function : Math  Operator=square  SaturateOnIntegerOverflow=on
  Mux : Mux  Inputs=3
  Mux1 : Mux  Inputs=10
  Mux2 : Mux  Inputs=3
  Sqrt : Sqrt  SaturateOnIntegerOverflow=on
  Sum of Elements : Sum  Inputs=+
  Trigonometric Function : Trigonometry  Operator=asin
  Trigonometric Function1 : Trigonometry  Operator=atan2
  x : Outport  VectorParamsAs1DForOutWhenUnconnected=off
  xdot : Outport  Port=2  VectorParamsAs1DForOutWhenUnconnected=off
  wires:
  Mux/1 -> xdot/1
  Compute Accel1/1(accel) -> Mux1/10  "hdd"
  Demux/5 -> Mux2/2, Trigonometric Function1/1, Mux/2
  Divide/1 -> Trigonometric Function/1
  Trigonometric Function1/1 -> Mux1/5, Compute Bank Angle/2(psi)  "psi"
  Trigonometric Function/1 -> Mux1/6  "theta"
  Compute Bank Angle/1(phi) -> Mux1/7  "phi"
  Compute Accel/1(accel) -> Mux1/8  "a"
  Mux1/1 -> x/1
  Sqrt/1 -> Divide/2, Mux1/1, Compute Bank Angle/1(speed), Compute Accel/1(speed)  "speed"
  Sum of Elements/1 -> Sqrt/1
  Math Function/1 -> Sum of Elements/1
  Mux2/1 -> Math Function/1
  Demux/6 -> Mux1/9, Compute Accel1/1(speed), Divide/1, Mux2/3, Mux/3  "hdot"
  Demux/4 -> Mux2/1, Trigonometric Function1/2, Mux/1
  Demux/3 -> Mux1/4  "Alt"
  Demux/2 -> Mux1/3  "E"
  Demux/1 -> Mux1/2  "N"
  From File/1 -> Demux/1

== system unitVisualAqSurveillance/AC2 - Track Following/Follow Trajectory/Null State Rate ==
  Bus Creator : BusCreator  Inputs='vdot_fpss','Ndot_ftps','Edot_ftps','hdot_ftps','psidot_radps','thetadot_radps','phidot_radps'  OutDataTypeStr=Bus: AircraftStateRate
  Constant{,1..6} (7 alike) : Constant  Value=0
  StateRate : Outport  OutDataTypeStr=Bus: AircraftStateRate  VectorParamsAs1DForOutWhenUnconnected=off
  wires:
  Constant6/1 -> Bus Creator/7  "phidot_radps"
  Constant5/1 -> Bus Creator/6  "thetadot_radps"
  Constant4/1 -> Bus Creator/5  "psidot_radps"
  Constant3/1 -> Bus Creator/4  "hdot_ftps"
  Constant2/1 -> Bus Creator/3  "Edot_ftps"
  Constant1/1 -> Bus Creator/2  "Ndot_ftps"
  Constant/1 -> Bus Creator/1  "vdot_fpss"
  Bus Creator/1 -> StateRate/1

== system unitVisualAqSurveillance/AC2 - Track Following/Follow Trajectory/Set LLA  ==
  State In : Inport
  Bus Assignment : BusAssignment  AssignedSignals=latLonAltState.lat_rad,latLonAltState.lon_rad,latLonAltState.dlat_radps,latLonAltState.dlon_radps,latLonAltState.alt_ft,latLonAltState.dalt_ftps
  Bus Selector : BusSelector  OutputSignals=e_ft,n_ft,h_ft,v_ftps,psi_rad,theta_rad
  Constant : Constant  Value=lat0
  Constant7 : Constant  Value=lon0
  Constant8 : Constant  Value=h0
  MATLAB Function : MATLAB Function  TreatAsAtomicUnit=on
  State Out : Outport  VectorParamsAs1DForOutWhenUnconnected=off
  wires:
  Bus Selector/6 -> MATLAB Function/6(theta_rad)  "<theta_rad>"
  Bus Selector/5 -> MATLAB Function/5(psi_rad)  "<psi_rad>"
  Bus Selector/4 -> MATLAB Function/4(v_ftps)  "<v_ftps>"
  Bus Selector/3 -> MATLAB Function/3(u_ft)  "<h_ft>"
  Bus Selector/2 -> MATLAB Function/2(n_ft)  "<n_ft>"
  Bus Selector/1 -> MATLAB Function/1(e_ft)  "<e_ft>"
  Constant8/1 -> MATLAB Function/9(h0)
  Constant7/1 -> MATLAB Function/8(lon0)
  Constant/1 -> MATLAB Function/7(lat0)
  State In/1 -> Bus Selector/1, Bus Assignment/1
  Bus Assignment/1 -> State Out/1
  MATLAB Function/6(dalt_ftps) -> Bus Assignment/7  "dalt_ftps"
  MATLAB Function/5(alt_ft) -> Bus Assignment/6  "alt_ft"
  MATLAB Function/4(dlon_radps) -> Bus Assignment/5  "dlon_radps"
  MATLAB Function/3(dlat_radps) -> Bus Assignment/4  "dlat_radps"
  MATLAB Function/2(lon_rad) -> Bus Assignment/3  "lon_rad"
  MATLAB Function/1(lat_rad) -> Bus Assignment/2  "lat_rad"

== system unitVisualAqSurveillance/AC2 - Track Following/Follow Trajectory/Set State ==
  x : Inport
  Bus Assignment : BusAssignment  AssignedSignals=v_ftps,n_ft,e_ft,h_ft,psi_rad,theta_rad,phi_rad,dv_ftps2,dh_ftps,ddh_ftps2
  Demux : Demux  Outputs=10
  Null AircraftState : Subsystem
  State : Outport  VectorParamsAs1DForOutWhenUnconnected=off
  wires:
  Demux/10 -> Bus Assignment/11
  Demux/9 -> Bus Assignment/10
  Bus Assignment/1 -> State/1
  Null AircraftState/1(State) -> Bus Assignment/1
  Demux/7 -> Bus Assignment/8  "phi"
  x/1 -> Demux/1
  Demux/6 -> Bus Assignment/7  "theta"
  Demux/5 -> Bus Assignment/6  "psi"
  Demux/4 -> Bus Assignment/5  "h"
  Demux/3 -> Bus Assignment/4  "E"
  Demux/2 -> Bus Assignment/3  "N"
  Demux/1 -> Bus Assignment/2  "v"
  Demux/8 -> Bus Assignment/9  "a"

== system unitVisualAqSurveillance/AC1 - Track Following/Follow Trajectory/Compute Body Rates/Compute p ==
  State : Inport
  Euler Rates : Inport  Port=2
  Add : Sum
  Bus Selector : BusSelector  OutputSignals=theta_rad
  Bus Selector1 : BusSelector  OutputSignals=psidot,phidot
  Product : Product
  Trigonometric Function : Trigonometry
  Unary Minus : UnaryMinus
  p : Outport  VectorParamsAs1DForOutWhenUnconnected=off
  wires:
  Add/1 -> p/1
  Unary Minus/1 -> Product/1
  Bus Selector1/2 -> Add/2  "<phidot>"
  Product/1 -> Add/1
  Trigonometric Function/1 -> Unary Minus/1
  State/1 -> Bus Selector/1
  Euler Rates/1 -> Bus Selector1/1
  Bus Selector/1 -> Trigonometric Function/1  "<theta_rad>"
  Bus Selector1/1 -> Product/2  "<psidot>"

== system unitVisualAqSurveillance/AC1 - Track Following/Follow Trajectory/Compute Body Rates/Compute q ==
  State : Inport
  Euler Rates : Inport  Port=2
  Add : Sum
  Bus Selector : BusSelector  OutputSignals=phi_rad,theta_rad
  Bus Selector1 : BusSelector  OutputSignals=thetadot,psidot
  Product : Product
  Product1 : Product  Inputs=3
  Trigonometric Function : Trigonometry  Operator=cos
  Trigonometric Function1 : Trigonometry  Operator=cos
  Trigonometric Function2 : Trigonometry
  q : Outport  VectorParamsAs1DForOutWhenUnconnected=off
  wires:
  Add/1 -> q/1
  Product1/1 -> Add/2
  Bus Selector1/2 -> Product1/3  "<psidot>"
  Trigonometric Function1/1 -> Product1/2
  Trigonometric Function2/1 -> Product1/1
  Bus Selector/2 -> Trigonometric Function1/1  "<theta_rad>"
  Bus Selector1/1 -> Product/2  "<thetadot>"
  Bus Selector/1 -> Trigonometric Function/1, Trigonometric Function2/1  "<phi_rad>"
  Trigonometric Function/1 -> Product/1
  Product/1 -> Add/1
  State/1 -> Bus Selector/1
  Euler Rates/1 -> Bus Selector1/1

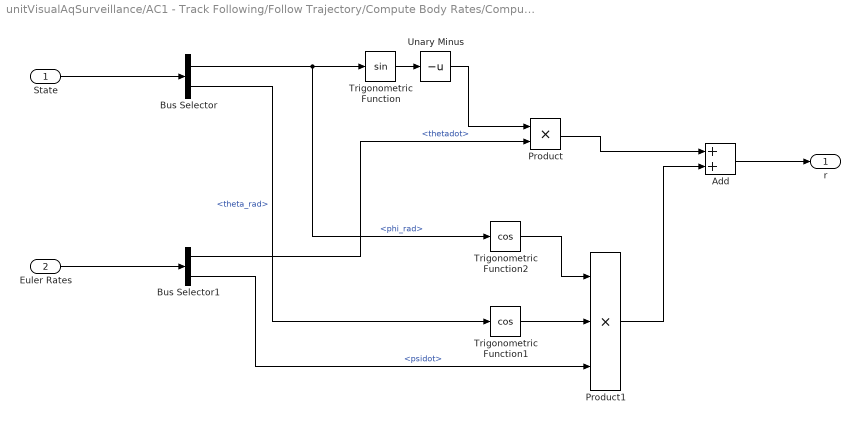
== system unitVisualAqSurveillance/AC1 - Track Following/Follow Trajectory/Compute Body Rates/Compute r ==
  State : Inport
  Euler Rates : Inport  Port=2
  Add : Sum
  Bus Selector : BusSelector  OutputSignals=phi_rad,theta_rad
  Bus Selector1 : BusSelector  OutputSignals=thetadot,psidot
  Product : Product
  Product1 : Product  Inputs=3
  Trigonometric Function : Trigonometry
  Trigonometric Function1 : Trigonometry  Operator=cos
  Trigonometric Function2 : Trigonometry  Operator=cos
  Unary Minus : UnaryMinus
  r : Outport  VectorParamsAs1DForOutWhenUnconnected=off
  wires:
  Unary Minus/1 -> Product/1
  Add/1 -> r/1
  Product1/1 -> Add/2
  Bus Selector1/2 -> Product1/3  "<psidot>"
  Trigonometric Function1/1 -> Product1/2
  Trigonometric Function2/1 -> Product1/1
  Bus Selector/2 -> Trigonometric Function1/1  "<theta_rad>"
  Bus Selector1/1 -> Product/2  "<thetadot>"
  Bus Selector/1 -> Trigonometric Function/1, Trigonometric Function2/1  "<phi_rad>"
  Trigonometric Function/1 -> Unary Minus/1
  Product/1 -> Add/1
  State/1 -> Bus Selector/1
  Euler Rates/1 -> Bus Selector1/1

== system unitVisualAqSurveillance/AC1 - Track Following/Follow Trajectory/Get Trajectory Data/Compute Accel ==
  speed : Inport
  Discrete Derivative : simulink/Discrete/Discrete Derivative  gainval=1.0  ICPrevScaledInput=0.0  OutMin=[]  OutMax=[]  OutDataType=fixdt(1, 16)  OutScaling=2^-10  DoSatur=off
  accel : Outport  VectorParamsAs1DForOutWhenUnconnected=off
  wires:
  Discrete Derivative/1 -> accel/1
  speed/1 -> Discrete Derivative/1

== system unitVisualAqSurveillance/AC1 - Track Following/Follow Trajectory/Get Trajectory Data/Compute Accel1 ==
  speed : Inport
  Discrete Derivative : simulink/Discrete/Discrete Derivative  gainval=1.0  ICPrevScaledInput=0.0  OutMin=[]  OutMax=[]  OutDataType=fixdt(1, 16)  OutScaling=2^-10  DoSatur=off
  accel : Outport  VectorParamsAs1DForOutWhenUnconnected=off
  wires:
  Discrete Derivative/1 -> accel/1
  speed/1 -> Discrete Derivative/1

== system unitVisualAqSurveillance/AC1 - Track Following/Follow Trajectory/Get Trajectory Data/Compute Bank Angle ==
  speed : Inport
  psi : Inport  Port=2
  Constant : Constant  Value=32.2
  Discrete Derivative : simulink/Discrete/Discrete Derivative  gainval=1.0  ICPrevScaledInput=0.0  OutMin=[]  OutMax=[]  OutDataType=fixdt(1, 16)  OutScaling=2^-10  DoSatur=off
  Divide : Product  Inputs=*/
  IC : InitialCondition  Value=0
  Product : Product
  Trigonometric Function : Trigonometry  Operator=atan
  phi : Outport  VectorParamsAs1DForOutWhenUnconnected=off
  wires:
  IC/1 -> Product/2
  Trigonometric Function/1 -> phi/1
  Divide/1 -> Trigonometric Function/1
  Constant/1 -> Divide/2
  Product/1 -> Divide/1
  psi/1 -> Discrete Derivative/1  "psi"
  speed/1 -> Product/1  "speed"
  Discrete Derivative/1 -> IC/1  "psidot"

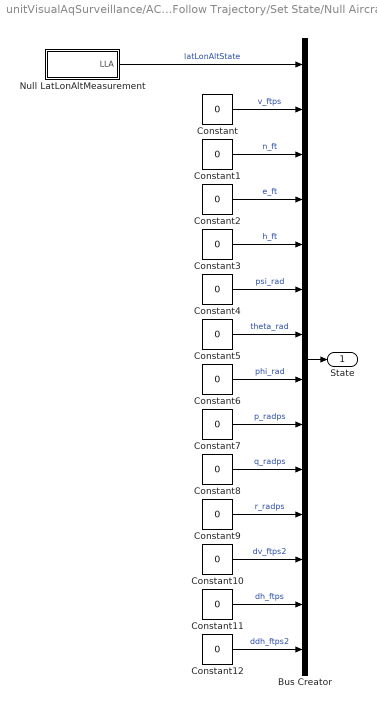
== system unitVisualAqSurveillance/AC1 - Track Following/Follow Trajectory/Set State/Null AircraftState ==
  Bus Creator : BusCreator  Inputs='latLonAltState','v_ftps','n_ft','e_ft','h_ft','psi_rad','theta_rad','phi_rad','p_radps','q_radps','r_radps','dv_ftps2','dh_ftps','ddh_ftps2'  OutDataTypeStr=Bus: AircraftState
  Constant{,1..12} (13 alike) : Constant  Value=0
  Null LatLonAltMeasurement : Subsystem
  State : Outport  VectorParamsAs1DForOutWhenUnconnected=off
  wires:
  Null LatLonAltMeasurement/1(LLA) -> Bus Creator/1  "latLonAltState"
  Constant/1 -> Bus Creator/2  "v_ftps"
  Constant12/1 -> Bus Creator/14  "ddh_ftps2"
  Constant1/1 -> Bus Creator/3  "n_ft"
  Bus Creator/1 -> State/1
  Constant6/1 -> Bus Creator/8  "phi_rad"
  Constant10/1 -> Bus Creator/12  "dv_ftps2"
  Constant7/1 -> Bus Creator/9  "p_radps"
  Constant5/1 -> Bus Creator/7  "theta_rad"
  Constant4/1 -> Bus Creator/6  "psi_rad"
  Constant8/1 -> Bus Creator/10  "q_radps"
  Constant9/1 -> Bus Creator/11  "r_radps"
  Constant3/1 -> Bus Creator/5  "h_ft"
  Constant2/1 -> Bus Creator/4  "e_ft"
  Constant11/1 -> Bus Creator/13  "dh_ftps"

== system unitVisualAqSurveillance/AC2 - Track Following/Follow Trajectory/Compute Body Rates/Compute p ==
  State : Inport
  Euler Rates : Inport  Port=2
  Add : Sum
  Bus Selector : BusSelector  OutputSignals=theta_rad
  Bus Selector1 : BusSelector  OutputSignals=psidot,phidot
  Product : Product
  Trigonometric Function : Trigonometry
  Unary Minus : UnaryMinus
  p : Outport  VectorParamsAs1DForOutWhenUnconnected=off
  wires:
  Add/1 -> p/1
  Unary Minus/1 -> Product/1
  Bus Selector1/2 -> Add/2  "<phidot>"
  Product/1 -> Add/1
  Trigonometric Function/1 -> Unary Minus/1
  State/1 -> Bus Selector/1
  Euler Rates/1 -> Bus Selector1/1
  Bus Selector/1 -> Trigonometric Function/1  "<theta_rad>"
  Bus Selector1/1 -> Product/2  "<psidot>"

== system unitVisualAqSurveillance/AC2 - Track Following/Follow Trajectory/Compute Body Rates/Compute q ==
  State : Inport
  Euler Rates : Inport  Port=2
  Add : Sum
  Bus Selector : BusSelector  OutputSignals=phi_rad,theta_rad
  Bus Selector1 : BusSelector  OutputSignals=thetadot,psidot
  Product : Product
  Product1 : Product  Inputs=3
  Trigonometric Function : Trigonometry  Operator=cos
  Trigonometric Function1 : Trigonometry  Operator=cos
  Trigonometric Function2 : Trigonometry
  q : Outport  VectorParamsAs1DForOutWhenUnconnected=off
  wires:
  Add/1 -> q/1
  Product1/1 -> Add/2
  Bus Selector1/2 -> Product1/3  "<psidot>"
  Trigonometric Function1/1 -> Product1/2
  Trigonometric Function2/1 -> Product1/1
  Bus Selector/2 -> Trigonometric Function1/1  "<theta_rad>"
  Bus Selector1/1 -> Product/2  "<thetadot>"
  Bus Selector/1 -> Trigonometric Function/1, Trigonometric Function2/1  "<phi_rad>"
  Trigonometric Function/1 -> Product/1
  Product/1 -> Add/1
  State/1 -> Bus Selector/1
  Euler Rates/1 -> Bus Selector1/1

== system unitVisualAqSurveillance/AC2 - Track Following/Follow Trajectory/Compute Body Rates/Compute r ==
  State : Inport
  Euler Rates : Inport  Port=2
  Add : Sum
  Bus Selector : BusSelector  OutputSignals=phi_rad,theta_rad
  Bus Selector1 : BusSelector  OutputSignals=thetadot,psidot
  Product : Product
  Product1 : Product  Inputs=3
  Trigonometric Function : Trigonometry
  Trigonometric Function1 : Trigonometry  Operator=cos
  Trigonometric Function2 : Trigonometry  Operator=cos
  Unary Minus : UnaryMinus
  r : Outport  VectorParamsAs1DForOutWhenUnconnected=off
  wires:
  Unary Minus/1 -> Product/1
  Add/1 -> r/1
  Product1/1 -> Add/2
  Bus Selector1/2 -> Product1/3  "<psidot>"
  Trigonometric Function1/1 -> Product1/2
  Trigonometric Function2/1 -> Product1/1
  Bus Selector/2 -> Trigonometric Function1/1  "<theta_rad>"
  Bus Selector1/1 -> Product/2  "<thetadot>"
  Bus Selector/1 -> Trigonometric Function/1, Trigonometric Function2/1  "<phi_rad>"
  Trigonometric Function/1 -> Unary Minus/1
  Product/1 -> Add/1
  State/1 -> Bus Selector/1
  Euler Rates/1 -> Bus Selector1/1

== system unitVisualAqSurveillance/AC2 - Track Following/Follow Trajectory/Get Trajectory Data/Compute Accel ==
  speed : Inport
  Discrete Derivative : simulink/Discrete/Discrete Derivative  gainval=1.0  ICPrevScaledInput=0.0  OutMin=[]  OutMax=[]  OutDataType=fixdt(1, 16)  OutScaling=2^-10  DoSatur=off
  accel : Outport  VectorParamsAs1DForOutWhenUnconnected=off
  wires:
  Discrete Derivative/1 -> accel/1
  speed/1 -> Discrete Derivative/1

== system unitVisualAqSurveillance/AC2 - Track Following/Follow Trajectory/Get Trajectory Data/Compute Accel1 ==
  speed : Inport
  Discrete Derivative : simulink/Discrete/Discrete Derivative  gainval=1.0  ICPrevScaledInput=0.0  OutMin=[]  OutMax=[]  OutDataType=fixdt(1, 16)  OutScaling=2^-10  DoSatur=off
  accel : Outport  VectorParamsAs1DForOutWhenUnconnected=off
  wires:
  Discrete Derivative/1 -> accel/1
  speed/1 -> Discrete Derivative/1

== system unitVisualAqSurveillance/AC2 - Track Following/Follow Trajectory/Get Trajectory Data/Compute Bank Angle ==
  speed : Inport
  psi : Inport  Port=2
  Constant : Constant  Value=32.2
  Discrete Derivative : simulink/Discrete/Discrete Derivative  gainval=1.0  ICPrevScaledInput=0.0  OutMin=[]  OutMax=[]  OutDataType=fixdt(1, 16)  OutScaling=2^-10  DoSatur=off
  Divide : Product  Inputs=*/
  IC : InitialCondition  Value=0
  Product : Product
  Trigonometric Function : Trigonometry  Operator=atan
  phi : Outport  VectorParamsAs1DForOutWhenUnconnected=off
  wires:
  IC/1 -> Product/2
  Trigonometric Function/1 -> phi/1
  Divide/1 -> Trigonometric Function/1
  Constant/1 -> Divide/2
  Product/1 -> Divide/1
  psi/1 -> Discrete Derivative/1  "psi"
  speed/1 -> Product/1  "speed"
  Discrete Derivative/1 -> IC/1  "psidot"

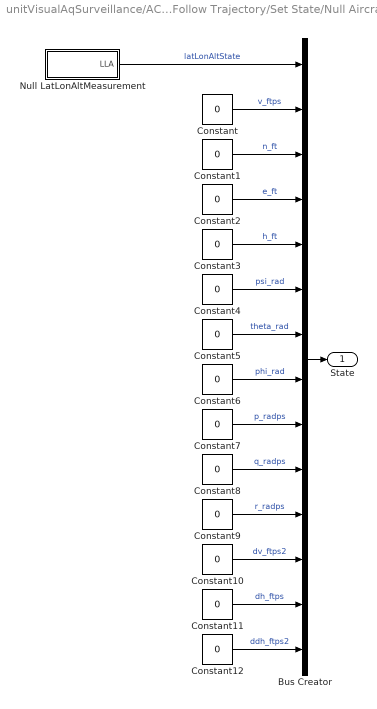
== system unitVisualAqSurveillance/AC2 - Track Following/Follow Trajectory/Set State/Null AircraftState ==
  Bus Creator : BusCreator  Inputs='latLonAltState','v_ftps','n_ft','e_ft','h_ft','psi_rad','theta_rad','phi_rad','p_radps','q_radps','r_radps','dv_ftps2','dh_ftps','ddh_ftps2'  OutDataTypeStr=Bus: AircraftState
  Constant{,1..12} (13 alike) : Constant  Value=0
  Null LatLonAltMeasurement : Subsystem
  State : Outport  VectorParamsAs1DForOutWhenUnconnected=off
  wires:
  Null LatLonAltMeasurement/1(LLA) -> Bus Creator/1  "latLonAltState"
  Constant/1 -> Bus Creator/2  "v_ftps"
  Constant12/1 -> Bus Creator/14  "ddh_ftps2"
  Constant1/1 -> Bus Creator/3  "n_ft"
  Bus Creator/1 -> State/1
  Constant6/1 -> Bus Creator/8  "phi_rad"
  Constant10/1 -> Bus Creator/12  "dv_ftps2"
  Constant7/1 -> Bus Creator/9  "p_radps"
  Constant5/1 -> Bus Creator/7  "theta_rad"
  Constant4/1 -> Bus Creator/6  "psi_rad"
  Constant8/1 -> Bus Creator/10  "q_radps"
  Constant9/1 -> Bus Creator/11  "r_radps"
  Constant3/1 -> Bus Creator/5  "h_ft"
  Constant2/1 -> Bus Creator/4  "e_ft"
  Constant11/1 -> Bus Creator/13  "dh_ftps"
